simulink model "slip"  (R2018b)
settings: Solver=ode4  StartTime=0.0  StopTime=10.0  FixedStep=0.01  RelTol=1e-3
settings Model: Creator=lpa1  LastModifiedBy=User

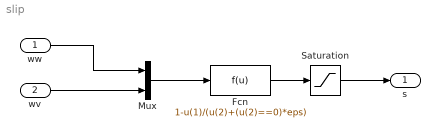
== system slip ==
  ww : Inport
  wv : Inport  Port=2
  Fcn : Fcn  Expr=1-u(1)/(u(2)+(u(2)==0)*eps)
  Mux : Mux  Inputs=2
  Saturation : Saturate  UpperLimit=1  LowerLimit=0
  s : Outport
  wires:
  Mux/1 -> Fcn/1
  ww/1 -> Mux/1
  wv/1 -> Mux/2
  Fcn/1 -> Saturation/1
  Saturation/1 -> s/1
